simulink model "B747_mpc_ss_du_restricoes"  (Simulink 7.9)
settings: Solver=ode4  SolverMode=SingleTasking  StartTime=0.0  StopTime=10  FixedStep=0.001  RelTol=1e-3
values from neighbouring files (symbols this model uses):
  Aqp = [eye(p*M);-eye(p*M);TMIp;-TMIp;G;-G]    [matrizes_ss_du_mimo_restricoes.m]
  Gn = Qbar*G    [matrizes_ss_du_mimo_restricoes.m]
  Hqp = 2*(G'*Qbar*G + Rbar)    [matrizes_ss_du_mimo_restricoes.m]
  Phi = [Phi;Ct*At^i]    [matrizes_ss_du_mimo_restricoes.m]
undefined symbols (not defined in the file or in its folder): A, Ac, B, Bc, C, T
settings Model: Creator=Kawakami  LastModifiedBy=Kawakami
settings DataIOCC: SignalLoggingName=sigsOut
settings OptimizationCC: BooleanDataType=off
settings DebuggingCC: SaveWithParameterizedLinksMsg=none  SignalResolutionControl=TryResolveAllWithWarning  SolverPrmCheckMsg=none  MultiTaskDSMMsg=warning  MultiTaskCondExecSysMsg=none  FcnCallInpInsideContextMsg=Use local settings  StrictBusMsg=None
settings HardwareCC: TargetUnknown=on
settings RTWCC: IncludeERTFirstTime=on
settings GRTTargetCC: CombineOutputUpdateFcns=off  GRTInterface=on

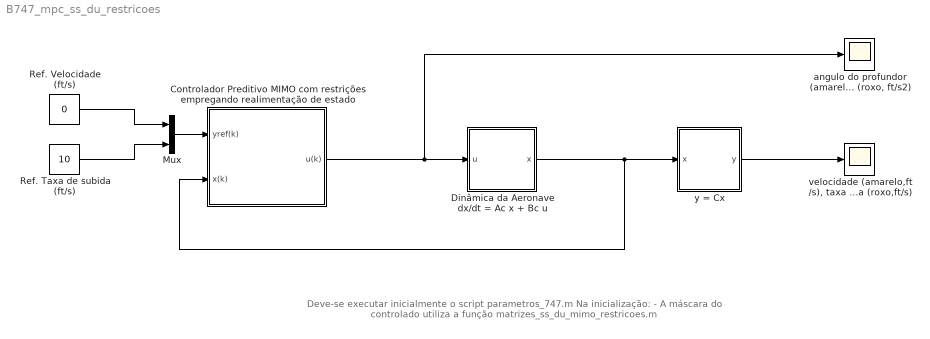
== system B747_mpc_ss_du_restricoes ==
  note: Deve-se executar inicialmente o script parametros_747.m
      |
      | Na inicialização:
      | - A máscara do controlado utiliza a função matrizes_ss_du_mimo_restricoes.m
  Controlador Preditivo MIMO com restrições empregando realimentação de estado : Subsystem  mask{rho=[1;1], mu=[1;1], N=20, M=10, A=A, B=B, C=C, dulim=[-inf inf;-inf inf], ulim=[-inf inf;-inf inf], ylim=[-inf inf;-inf inf], T=T}
      mask prompts: rho "Pesos dos controle (rho) (p x 1)"; mu "Pesos das saídas mu (q x 1)"; N "Horizonte de Predição (N)"; M "Horizonte de Controle (M)"; A "Matriz A (n x n)"; B "Matriz B (n x p)"; C "Matriz C (q x n)"; dulim "[dumin, dumax] (p x 2)"; ulim "[umin, umax] (p x 2)"; ylim "[ymin, ymax] (q x 2)"; T "Periodo de amostragem"
      mask init:
      | [Phi,Gn,Hqp,Aqp] = matrizes_ss_du_mimo_restricoes(A,B,C,N,M,mu,rho);
      | n = size(A,1);
      | p = size(B,2);
      | q = size(C,1);
      | umin = ulim(:,1);
      | umax = ulim(:,2);
      | dumin = dulim(:,1);
      | dumax = dulim(:,2);
      | ymin = ylim(:,1);
      | ymax = ylim(:,2);
  Dinâmica da Aeronave dx/dt = Ac x + Bc u : Subsystem
  Mux : Mux  Inputs=2
  Ref. Taxa de subida (ft/s) : Constant  Value=10
  Ref. Velocidade (ft/s) : Constant  Value=0
  "angulo do profundor (amarelo, crad) tração específica (roxo, ft/s2)" : Scope
      settings: TimeRange=10  YMax=3  SaveName=y1
  "velocidade (amarelo,ft/s), taxa de subida (roxo,ft/s)" : Scope
      settings: TimeRange=10  YMin=-2  YMax=12  SaveName=y
  y = Cx : Subsystem
  wires:
  Controlador Preditivo MIMO com restrições empregando realimentação de estado/1(u(k)) -> "angulo do profundor (amarelo, crad) tração específica (roxo, ft/s2)"/1, Dinâmica da Aeronave dx/dt = Ac x + Bc u/1(u)
  Dinâmica da Aeronave dx/dt = Ac x + Bc u/1(x) -> y = Cx/1(x), Controlador Preditivo MIMO com restrições empregando realimentação de estado/2(x(k))
  Mux/1 -> Controlador Preditivo MIMO com restrições empregando realimentação de estado/1(yref(k))
  Ref. Velocidade (ft/s)/1 -> Mux/1
  Ref. Taxa de subida (ft/s)/1 -> Mux/2
  y = Cx/1(y) -> "velocidade (amarelo,ft/s), taxa de subida (roxo,ft/s)"/1

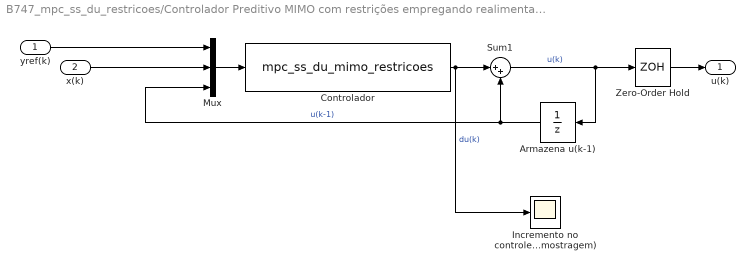
== system B747_mpc_ss_du_restricoes/Controlador Preditivo MIMO com restrições empregando realimentação de estado ==
  yref(k) : Inport
  x(k) : Inport  Port=2
  Armazena u(k-1) : UnitDelay  SampleTime=T
  Controlador : S-Function  FunctionName=mpc_ss_du_mimo_restricoes  Parameters=Phi,Gn,Hqp,Aqp,dumax,dumin,umax,umin,ymax,ymin,p,q,n,M,N,T  EnableBusSupport=off
  Incremento no controle du (volts/período de amostragem) : Scope
      settings: TimeRange=2  YMin=-0.3  YMax=0.2
  Mux : Mux  Inputs=3
  Sum1 : Sum  Inputs=|++  SaturateOnIntegerOverflow=on  InputSameDT=on  OutDataTypeStr=Inherit: Same as first input
  Zero-Order Hold : ZeroOrderHold  SampleTime=T
  u(k) : Outport
  wires:
  Mux/1 -> Controlador/1
  Zero-Order Hold/1 -> u(k)/1
  x(k)/1 -> Mux/2
  yref(k)/1 -> Mux/1
  Sum1/1 -> Zero-Order Hold/1, Armazena u(k-1)/1  "u(k)"
  Armazena u(k-1)/1 -> Sum1/2, Mux/3  "u(k-1)"
  Controlador/1 -> Sum1/1, Incremento no controle du (volts/período de amostragem)/1  "du(k)"

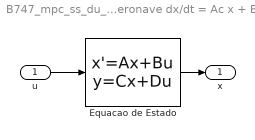
== system B747_mpc_ss_du_restricoes/Dinâmica da Aeronave dx/dt = Ac x + Bc u ==
  u : Inport
  Equacao de Estado : StateSpace  A=Ac  B=Bc  C=eye(size(A,1),size(A,1))  D=zeros(size(A,1),size(B,2))  X0=zeros(size(A,1),1)
  x : Outport
  wires:
  u/1 -> Equacao de Estado/1
  Equacao de Estado/1 -> x/1

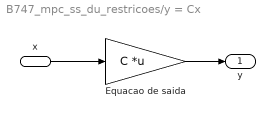
== system B747_mpc_ss_du_restricoes/y = Cx ==
  x : Inport
  Equacao de saida : Gain  Gain=C  Multiplication=Matrix(K*u)  SaturateOnIntegerOverflow=on  OutDataTypeStr=Inherit: Same as input  ParamDataTypeStr=Inherit: Same as input
  y : Outport
  wires:
  x/1 -> Equacao de saida/1
  Equacao de saida/1 -> y/1
